simulink model "modelo_quad13_ver76"  (Simulink 8.3)
settings: Solver=ode45  StartTime=0.0  StopTime=100  FixedStep=0.025  MaxStep=0.1  RelTol=1e-3
values from neighbouring files (symbols this model uses):
  accel_noise = 0    [main_quad.m]
  baccx = 1e-1    (= 0.1)    [main_quad.m]
  baccy = 1e-1    (= 0.1)    [main_quad.m]
  baccz = 1e-1    (= 0.1)    [main_quad.m]
  baro_noise = 0    [main_quad.m]
  bgyrp = 1e-3    (= 0.001)    [main_quad.m]
  bgyrq = 1e-3    (= 0.001)    [main_quad.m]
  bgyrr = 1e-3    (= 0.001)    [main_quad.m]
  bmagx = 1e-6    (= 1e-06)    [main_quad.m]
  bmagy = -1e-6    (= -1e-06)    [main_quad.m]
  bmagz = 1e-6    (= 1e-06)    [main_quad.m]
  controle = 0    [main_quad.m]
  correct_acc = 1    [main_quad.m]
  cq = 2.4086*10^(-7)    (= 2.4086e-07)    [main_quad.m]
  cq_real = cq    (= 2.4086e-07)    [main_quad.m]
  ct = 1.4341*10^(-5)    (= 1.4341e-05)    [main_quad.m]
  ct_real = ct    (= 1.4341e-05)    [main_quad.m]
  d = 0.26    [main_quad.m]
  g = 9.8065    [main_quad.m]
  gps_noise_on = 0    [main_quad.m]
  gyro_noise = 0    [main_quad.m]
  J = [Jxx,Jyy,Jzz,Jm]    [main_quad.m]
  J_real = J    [main_quad.m]
  Ja = 5e-5    (= 5e-05)    [main_quad.m]
  k1 = 2.5    [main_quad.m]
  k2 = 6.2360    (= 6.236)    [main_quad.m]
  k3 = 6.2360    (= 6.236)    [main_quad.m]
  k4 = 0.4927    [main_quad.m]
  k5 = 1.6    [main_quad.m]
  k6 = 1.6    [main_quad.m]
  ke = kt    (= 0.024)    [main_quad.m]
  kt = 0.024    [main_quad.m]
  lambda1 = 1    [main_quad.m]
  lambda2 = 5    [main_quad.m]
  lambda3 = 5    [main_quad.m]
  lambda4 = 1/2    (= 0.5)    [main_quad.m]
  lambda5 = 1/4    (= 0.25)    [main_quad.m]
  lambda6 = 1/4    (= 0.25)    [main_quad.m]
  limit = [0.5 0.5 0.5 0.5]    [main_quad.m]
  limit_pos = [0.5 0.5]    [main_quad.m]
  m = 1.03    [main_quad.m]
  m_real = m    (= 1.03)    [main_quad.m]
  mag_noise = 0    [main_quad.m]
  max_w = 733.03    [main_quad.m]
  mgeo = [17223.7  -4581.6 -13698.2 ]'*1e-9    [main_quad.m]
  p0 = 0    [main_quad.m]
  phi0 = 0    [main_quad.m]
  Pitch_D = 0.019    [main_quad.m]
  Pitch_P = 0.019948    [main_quad.m]
  pos_D = -0.033991    [main_quad.m]
  pos_P = -0.005948    [main_quad.m]
  psi0 = 0    [main_quad.m]
  q0 = 0    [main_quad.m]
  R = 0.2    [main_quad.m]    (also in plot_resultados.m = A(:,12))
  r0 = 0    [main_quad.m]
  Roll_D = 0.019    [main_quad.m]
  Roll_P = 0.019948    [main_quad.m]
  t_d = 50e-3    (= 0.05)    [main_quad.m]
  theta0 = 0    [main_quad.m]
  Tnoise_gps = TsGPS    (= 0.2)    [main_quad.m]
  Ts_bar = 0.1    [main_quad.m]
  TsGPS = 1/fGPS    (= 0.2)    [main_quad.m]
  Tsr = 1e-2    (= 0.01)    [main_quad.m]
  vx0 = 0    [main_quad.m]
  vy0 = 0    [main_quad.m]
  vz0 = 0    [main_quad.m]
  w1_0 = w_hover    [main_quad.m]
  w2_0 = w_hover    [main_quad.m]
  w3_0 = w_hover    [main_quad.m]
  w4_0 = w_hover    [main_quad.m]
  w_f_gps = 2*pi*(2*fGPS)    (= 62.8318530718)    [main_quad.m]
  w_f_triad = 2*pi*(10)    (= 62.8318530718)    [main_quad.m]
  x0 = 0    [main_quad.m]
  y0 = 0    [main_quad.m]
  Yaw_D = 0.037200    (= 0.0372)    [main_quad.m]
  Yaw_P = 0.039055    [main_quad.m]
  z0 = 0    [main_quad.m]
  Z_D = -0.682000    (= -0.682)    [main_quad.m]
  Z_P = -0.238672    [main_quad.m]
libraries: simulink x18
(part 2 of 2)

== matlab function Controle/Controlador PD/Controle de Translação/Controle de Posição/conversao ref. angulos ==
  data: ux input double; uy input double; psi input double; phi input double; phi_ref output double; theta_ref output double
function [phi_ref,theta_ref] = conv_ang_ref(ux,uy,psi,phi)

arg_phi = ux*sin(psi)-uy*cos(psi);

if arg_phi>1
    arg_phi=1;
elseif arg_phi<-1
    arg_phi=-1;
end

arg_theta = (ux*cos(psi)+uy*sin(psi))/(cos(phi));

if arg_theta>1
    arg_theta=1;
elseif arg_theta<-1
    arg_theta=-1;
end


phi_ref = asin(arg_phi);

theta_ref = asin(arg_theta);

== matlab function Controle/Controlador sliding mode/MATLAB Function ==
  data: u_T output double; u_L output double; g input double; J input double; m input double; Phi input double; Theta input double; Psi input double; y input double; y_dot input double; yd input double; yd_dot input double; yd_dotdot input double; lambda input double; k input double; u_M output double; u_N output double; limit input double; s output double
function [u_T,u_L,u_M,u_N,s] = sliding_mode(g,J,m,Phi,Theta,Psi,y,y_dot,yd,yd_dot,yd_dotdot,lambda,k, limit)

Jxx=J(1);
Jyy=J(2);
Jzz=J(3);

lambdas = [lambda(1),0,0,0
          0,lambda(2),0,0
          0,0,lambda(3),0
          0,0,0,lambda(4)];

Phid = y_dot(2);
Thetad = y_dot(3);
Psid = y_dot(4);
      
f=zeros(4,1);

f(1)= g;

f(2)= cos(Phi)*tan(Theta)*(((Phid - Psid*sin(Theta))*(Jxx - Jyy)*(Thetad*cos(Phi) + ...
Psid*cos(Theta)*sin(Phi)))/Jzz) + sin(Phi)*tan(Theta)*(((Phid - Psid*sin(Theta))*(Jxx - Jzz)*(Thetad*sin(Phi) - Psid*cos(Phi)*cos(Theta)))/Jyy) + ...
(Psid*Thetad)/cos(Theta) + Phid*Thetad*tan(Theta) - ((Jyy - Jzz)*(Thetad*cos(Phi) + Psid*cos(Theta)*sin(Phi))*(Thetad*sin(Phi) - Psid*cos(Phi)*cos(Theta)))/Jxx;

f(3)= cos(Phi)*(((Phid - Psid*sin(Theta))*(Jxx - Jzz)*(Thetad*sin(Phi) - Psid*cos(Phi)*cos(Theta)))/Jyy) +...
    - sin(Phi)*(((Phid - Psid*sin(Theta))*(Jxx - Jyy)*(Thetad*cos(Phi) + Psid*cos(Theta)*sin(Phi)))/Jzz) - Phid*Psid*cos(Theta);

f(4) = (Phid*Thetad)/cos(Theta) + (cos(Phi)*(Jxx*(Phid - Psid*sin(Theta))*(Thetad*cos(Phi) + Psid*cos(Theta)*sin(Phi)) - Jyy*(Phid - Psid*sin(Theta))*(Thetad*cos(Phi) + Psid*cos(Theta)*sin(Phi))))/(Jzz*cos(Theta)) + ...
(sin(Phi)*(Jxx*(Phid - Psid*sin(Theta))*(Thetad*sin(Phi) - Psid*cos(Phi)*cos(Theta)) - Jzz*(Phid - Psid*sin(Theta))*(Thetad*sin(Phi) - Psid*cos(Phi)*cos(Theta))))/(Jyy*cos(Theta)) + (Psid*Thetad*sin(Theta))/cos(Theta);

s = y_dot - yd_dot + lambdas*(y - yd);


Binv=[-m/(cos(Phi)*cos(Theta)),0,0,0
       0, Jxx, 0,  -Jxx*sin(Theta)
       0, 0, (Jyy*cos(Phi)), (Jyy*cos(Theta)*sin(Phi))
       0, 0, -(Jzz*sin(Phi)), (Jzz*cos(Phi)*cos(Theta))];

k_des =  [k(1),0,0,0
          0,k(2),0,0
          0,0,k(3),0
          0,0,0,k(4)];
 
u = Binv * (-f + yd_dotdot - lambdas*(y_dot - yd_dot) - k_des * sat(s,limit));


u_T = u(1);
u_L = u(2);
u_M = u(3);
u_N = u(4);

== matlab function Controle/Controlador sliding mode/MATLAB Function1 ==
  data: p input double; phi_dot output double; q input double; r input double; phi input double; theta input double; psi input double; theta_dot output double; psi_dot output double
function [phi_dot,theta_dot,psi_dot] = pqr_to_euler_dot(p,q,r,phi,theta,psi)

phi_dot = p + tan(theta)*sin(phi)*q + tan(theta)*cos(phi)*r;

theta_dot = cos(phi)*q - sin(phi)*r;

psi_dot = q*sin(phi)/cos(theta) + r*cos(phi)/cos(theta);

== matlab function Controle/Controlador sliding mode/Controle de Translação/conversao ref. angulos ==
  data: ux input double; uy input double; psi input double; phi input double; phi_ref output double; theta_ref output double
function [phi_ref,theta_ref] = conv_ang_ref(ux,uy,psi,phi)

arg_phi = ux*sin(psi)-uy*cos(psi);

if arg_phi>1
    arg_phi=1;
elseif arg_phi<-1
    arg_phi=-1;
end

arg_theta = (ux*cos(psi)+uy*sin(psi))/(cos(phi));

if arg_theta>1
    arg_theta=1;
elseif arg_theta<-1
    arg_theta=-1;
end


phi_ref = asin(arg_phi);

theta_ref = asin(arg_theta);

== matlab function Controle/Controlador sliding mode/Controle de Translação/MATLAB Function ==
  data: m input double; T input double; lambda input double; k input double; y input double; y_dot input double; yd input double; yd_dot input double; yd_dotdot input double; ux output double; uy output double; limit input double
function [ux,uy] = posicao_sliding(m,T,lambda, k, y, y_dot, yd, yd_dot, yd_dotdot, limit)

lambdas=[lambda(1), 0
            0, lambda(2)];
        
k_des = [ k(1), 0 
             0, k(2)];
         
Binv= [-m/T, 0
        0, -m/T];
    
s = y_dot - yd_dot + lambdas*(y - yd);

u = Binv*(yd_dotdot - lambdas*(y_dot-yd_dot) - k_des*sat(s,limit));

ux=u(1);
uy=u(2);

== matlab function sensores/TRIAD3/Embedded MATLAB Function ==
  data: ab input double size=[3,1]; phi output double size=[1,1]; mb input double size=[3,1]; ar input double size=[3,1]; mr input double size=[3,1]; theta output double size=[1,1]; psi output double size=[1,1]
function [phi,theta,psi]=TRIADT3(ab,mb,ar,mr)
%#eml

% Normalizacao dos vetores
ab=ab/norm(ab); % gravidade no corpo
b1=ab;
mb=mb/norm(mb); % vetor geomagnetico no corpo
b2=mb;

ar=ar/norm(ar); % gravidade na referencia
r1=ar;
mr=mr/norm(mr); % vetor geomagnetico na referencia
r2=mr;

% Vetores mais e menos
b_mais=(b2+b1)/norm(b2+b1);
b_menos=(b2-b1)/norm(b2-b1);

r_mais=(r1+r2)/norm(r1+r2);
r_menos=(r2-r1)/norm(r2-r1);

% Terceiro vetor
b3=cross(b_mais,b_menos)/norm(cross(b_mais,b_menos)); % terceiro vetor no corpo

r3=cross(r_mais,r_menos)/norm(cross(r_mais,r_menos)); % terceiro vetor na referencia

% Calculo da matriz de atitude numero 3
AT3=b_mais*r_mais'+b_menos*r_menos'+b3*r3';

% Conversao da matriz de atitude (matriz de cossenos diretores) para
% angulos de Euler na Rotacao Z-Y-X
[phi,theta,psi]=mat2euler(AT3);
